simulink model "pidtune_demo"  (Simulink 6.0)
settings: Solver=ode23t  StartTime=0.0  StopTime=20  RelTol=0.001
PreLoadFcn:
  | load pidtune_demo
undefined symbols (not defined in the file or in its folder): Kd, Ki, Kp
libraries: srolib x2
settings Model: Creator=ksubbara  LastModifiedBy=pascal  ModelDataFile=srodemo1.mat
settings DataIOCC: SaveOutput=off  SaveTime=off  SignalLoggingName=sigsOut
settings DebuggingCC: CheckExecutionContextPreStartOutputMsg=on  CheckExecutionContextRuntimeOutputMsg=on  SolverPrmCheckMsg=none
settings HardwareCC: TargetUnknown=on
settings ModelReferenceCC: UpdateModelReferenceTargets=IfOutOfDate
settings GRTTargetCC: LifeSpan=inf
settings SFSimCC: SFSimApplyToAllLibs=on  SFSimBuildMode=Incremental

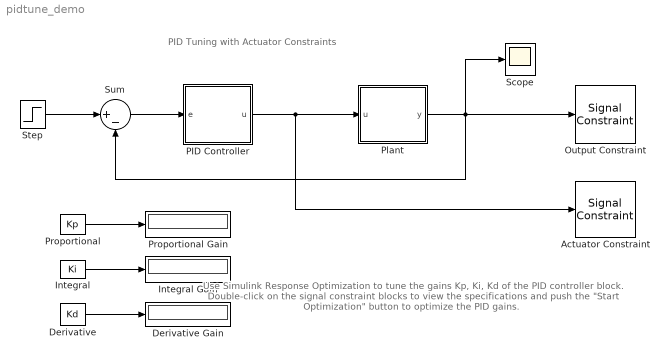
== system pidtune_demo ==
  note: Use Simulink Response Optimization to
      | tune the gains Kp, Ki, Kd of the
      | PID controller block.
      |
      | Double-click on the signal constraint blocks to
      | view the specifications and push the "Start Optimization"
      | button to optimize the PID gains.
  note: PID Tuning with Actuator Constraints
  Actuator Constraint : srolib/Signal Constraint  DialogPosition=[0.401875 0.274166666666667 0.36125 0.261666666666667]  SaveIn=workspace  SaveAs=pidtune_optim  LogID=SRO_DataLog_1
  Derivative : Constant  Value=Kd
  Derivative Gain : Display
  Integral : Constant  Value=Ki
  Integral Gain : Display
  Output Constraint : srolib/Signal Constraint  DialogPosition=[0.058125 0.273333333333333 0.33875 0.26]  SaveIn=workspace  SaveAs=pidtune_optim  LogID=SRO_DataLog_2
  PID Controller : Subsystem  PropExecContextAcrossSSBoundary=on
  Plant : Subsystem  PropExecContextAcrossSSBoundary=on
  Proportional : Constant  Value=Kp
  Proportional Gain : Display
  Scope : Scope
  Step : Step  Time=0.01  SampleTime=0
  Sum : Sum  Inputs=|+-  SaturateOnIntegerOverflow=on
  wires:
  Sum/1 -> PID Controller/1(e)
  Step/1 -> Sum/1
  PID Controller/1(u) -> Plant/1("u "), Actuator Constraint/1
  Proportional/1 -> Proportional Gain/1
  Integral/1 -> Integral Gain/1
  Derivative/1 -> Derivative Gain/1
  Plant/1(y) -> Sum/2, Scope/1, Output Constraint/1

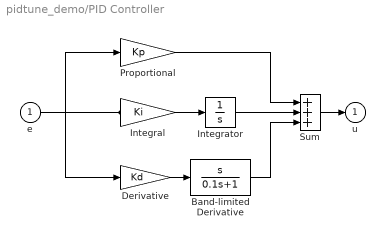
== system pidtune_demo/PID Controller ==
  e : Inport  LatchInput=off
  Band-limited Derivative : TransferFcn  Numerator=[1 0]  Denominator=[0.1 1]
  Derivative : Gain  Gain=Kd  SaturateOnIntegerOverflow=on
  Integral : Gain  Gain=Ki  SaturateOnIntegerOverflow=on
  Integrator : Integrator
  Proportional : Gain  Gain=Kp  SaturateOnIntegerOverflow=on
  Sum : Sum  Inputs=+++  SaturateOnIntegerOverflow=on  InputSameDT=on
  u : Outport  InitialOutput=0
  wires:
  Proportional/1 -> Sum/1
  Integral/1 -> Integrator/1
  Band-limited Derivative/1 -> Sum/3
  e/1 -> Derivative/1, Proportional/1, Integral/1
  Sum/1 -> u/1
  Derivative/1 -> Band-limited Derivative/1
  Integrator/1 -> Sum/2

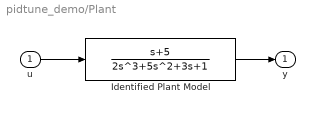
== system pidtune_demo/Plant ==
  "u " : Inport  LatchInput=off
  Identified Plant Model : TransferFcn  Numerator=[1 5]  Denominator=[2 5 3 1]
  y : Outport  InitialOutput=0
  wires:
  Identified Plant Model/1 -> y/1
  "u "/1 -> Identified Plant Model/1
